simulink model "Navion_6DoF_YANG"  (Simulink 10.3)
settings: Solver=ode45  StartTime=0.0  StopTime=100.0  FixedStep=.01  MaxStep=.004  RelTol=1e-5  EnableMultiTasking=on
values from neighbouring files (symbols this model uses):
  ac = [0 0 0]    [Navion_Geom6dof.m]
  b = 44    [Navion_Geom6dof.m]
  cbar = 4+2/12    (= 4.16666666667)    [Navion_Geom6dof.m]
  cda2 = 0.33    [Navion_Geom6dof.m]
  cdo = 0.05    [Navion_Geom6dof.m]
  cg = [0 0 0]    [Navion_Geom6dof.m]
  cla = 4.44    [Navion_Geom6dof.m]
  cladot = 0    [Navion_Geom6dof.m]
  clb = -0.074    [Navion_Geom6dof.m]
  clda = -0.134    [Navion_Geom6dof.m]
  clde = 0.355    [Navion_Geom6dof.m]
  cldr = 0.107    [Navion_Geom6dof.m]
  clo = 0.41    [Navion_Geom6dof.m]
  clp = -0.410    (= -0.41)    [Navion_Geom6dof.m]
  clq = 3.8    [Navion_Geom6dof.m]
  clr = 0.107    [Navion_Geom6dof.m]
  cma = -0.683    [Navion_Geom6dof.m]
  cmadot = -4.36    [Navion_Geom6dof.m]
  cmde = -0.923    [Navion_Geom6dof.m]
  cmq = -9.96    [Navion_Geom6dof.m]
  cnb = 0.071    [Navion_Geom6dof.m]
  cnda = -0.0035    [Navion_Geom6dof.m]
  cndr = -0.072    [Navion_Geom6dof.m]
  cnp = -0.0575    [Navion_Geom6dof.m]
  cnr = -0.125    [Navion_Geom6dof.m]
  cyb = -0.564    [Navion_Geom6dof.m]
  cydr = 0.157    [Navion_Geom6dof.m]
  initalt = 6000    [Navion_Geom6dof.m]
  initbank = 0    [Navion_Geom6dof.m]
  initeast = 0    [Navion_Geom6dof.m]
  inithead = 0    [Navion_Geom6dof.m]
  initnorth = 0    [Navion_Geom6dof.m]
  initp = 0    [Navion_Geom6dof.m]
  initpitch = initw/initu    (= -0.0290599038041)    [Navion_Geom6dof.m]
  initq = 0    [Navion_Geom6dof.m]
  initr = 0    [Navion_Geom6dof.m]
  initu = 228.7    [Navion_Geom6dof.m]
  initv = 0    [Navion_Geom6dof.m]
  initw = -6.646    [Navion_Geom6dof.m]
  jx = 1048    [Navion_Geom6dof.m]
  jxz = 0    [Navion_Geom6dof.m]
  jy = 3000    [Navion_Geom6dof.m]
  jz = 3500    [Navion_Geom6dof.m]
  Pos_L = [95.46/12-3.882,5.1875,0]    [Navion_Geom6dof.m]
  Pos_R = [95.46/12,-5.1875,0]    [Navion_Geom6dof.m]
  sw = 175.3    [Navion_Geom6dof.m]
  Vect_L = [0.998,-0.057,0.017]    [Navion_Geom6dof.m]
  Vect_R = [0.998,0.057,0.017]    [Navion_Geom6dof.m]
  weight = 3695    [Navion_Geom6dof.m]
undefined symbols (not defined in the file or in its folder): BHP_A, BHP_B, CP_norm, Pr_Alt, PropEff_norm
libraries: simulink_extras x4, aerolibatmos2 x2
(part 2 of 2)

== system Navion_6DoF_YANG/Aircraft_Dynamics/Aerodynamics/Aero Forces and Moments/Aerodynamic Forces/Body to Wind ==
  note: This transforms any arbitrary vector from body axis to wind axis.
      | Page 63  Stevens and Lewis
  Alpha : Inport
  Beta : Inport  Port=2
  -ca sb : Fcn  Expr=-1 * cos(u[1]) * sin(u[2])
  -sa : Fcn  Expr=-1 * sin(u[1])
  -sa sb : Fcn  Expr="-1 * sin(u[1])  * sin(u[2])"
  Fcn8 : Fcn  Expr=cos(u[1])
  Matrix Concatenation : Concatenate  NumInputs=3  Mode=Multidimensional array
  Matrix Concatenation1 : Concatenate  NumInputs=3  Mode=Multidimensional array
  Matrix Concatenation2 : Concatenate  NumInputs=3  Mode=Multidimensional array  ConcatenateDimension=2
  Matrix Concatenation3 : Concatenate  NumInputs=3  Mode=Multidimensional array
  Mux1 : Mux  Inputs=2
  ca cb : Fcn  Expr="cos(u[1]) *  cos(u[2])"
  cb : Fcn  Expr=cos(u[2])
  sa cb : Fcn  Expr=sin(u[1]) * cos(u[2])
  sb : Fcn  Expr=sin(u[2])
  zero : Fcn  Expr=u[1] * 0
  Smatrix : Outport
  wires:
  Matrix Concatenation/1 -> Matrix Concatenation2/1
  Matrix Concatenation1/1 -> Matrix Concatenation2/2
  Matrix Concatenation3/1 -> Matrix Concatenation2/3
  -ca sb/1 -> Matrix Concatenation/2
  ca cb/1 -> Matrix Concatenation/1
  -sa/1 -> Matrix Concatenation/3
  zero/1 -> Matrix Concatenation1/3
  sb/1 -> Matrix Concatenation1/1
  cb/1 -> Matrix Concatenation1/2
  sa cb/1 -> Matrix Concatenation3/1
  -sa sb/1 -> Matrix Concatenation3/2
  Fcn8/1 -> Matrix Concatenation3/3
  Mux1/1 -> ca cb/1, -ca sb/1, -sa/1, sb/1, cb/1, zero/1, sa cb/1, -sa sb/1, Fcn8/1
  Alpha/1 -> Mux1/1
  Beta/1 -> Mux1/2
  Matrix Concatenation2/1 -> Smatrix/1

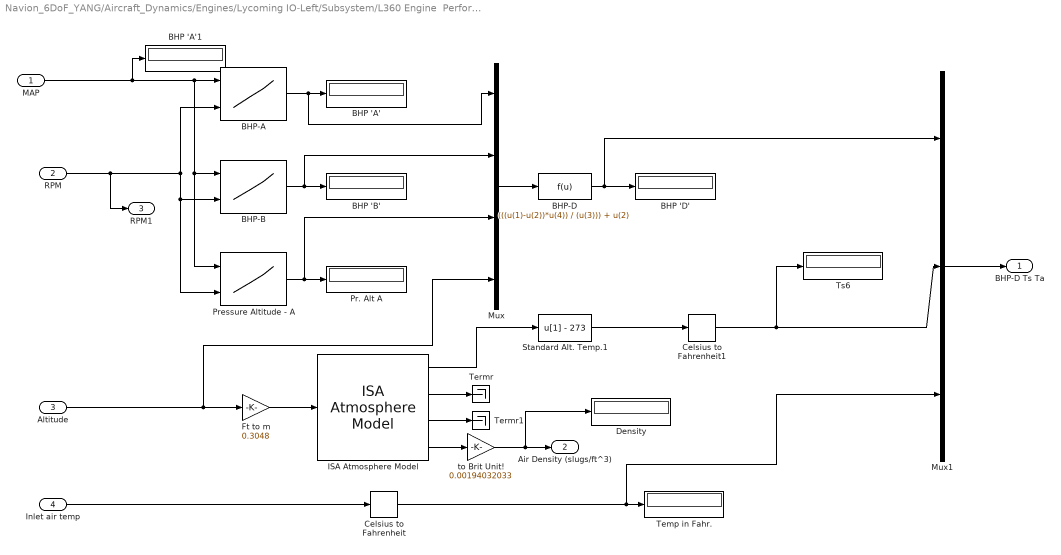
== system Navion_6DoF_YANG/Aircraft_Dynamics/Engines/Lycoming IO-Left/Subsystem/L360 Engine  Performance Data ==
  MAP : Inport
  RPM : Inport  Port=2
  Altitude : Inport  Port=3
  Inlet air temp : Inport  Port=4
  BHP 'A' : Display
  BHP 'A'1 : Display
  BHP 'B' : Display
  BHP 'D' : Display
  BHP-A : Lookup2D  RowIndex=MAP  ColumnIndex=RPM  Table=BHP_A  LookUpMeth=Interpolation-Use End Values
  BHP-B : Lookup2D  RowIndex=MAP  ColumnIndex=RPM  Table=BHP_B  LookUpMeth=Interpolation-Use End Values
  BHP-D : Fcn  Expr=(((u(1)-u(2))*u(4)) / (u(3))) + u(2)
  Celsius to Fahrenheit : simulink_extras/Transformations/Celsius to Fahrenheit
      settings: SourceProductBaseCode=SL
  Celsius to Fahrenheit1 : simulink_extras/Transformations/Celsius to Fahrenheit
      settings: SourceProductBaseCode=SL
  Density : Display
  Ft to m : Gain  Gain=0.3048
  ISA Atmosphere Model : aerolibatmos2/ISA Atmosphere Model  custom=off  g=9.80665  gamma=1.4  R=287.0531  L=0.0065  h_trop=11000  h_strat=20000  rho0=1.225  P0=101325  T0=288.15  h0=0
  Mux : Mux
  Mux1 : Mux  Inputs=3
  Pr. Alt A : Display
  Pressure Altitude - A : Lookup2D  RowIndex=MAP  ColumnIndex=RPM  Table=Pr_Alt  LookUpMeth=Interpolation-Use End Values
  Standard Alt. Temp.1 : Fcn  Expr=u[1] - 273
  Temp in Fahr. : Display
  Termr : Terminator
  Termr1 : Terminator
  Ts6 : Display
  to Brit Unit! : Gain  Gain=0.00194032033
  BHP-D Ts Ta : Outport
  Air Density (slugs/ft^3) : Outport  Port=2
  RPM1 : Outport  Port=3
  wires:
  MAP/1 -> BHP 'A'1/1, Pressure Altitude - A/1, BHP-B/1, BHP-A/1
  ISA Atmosphere Model/1 -> Standard Alt. Temp.1/1
  to Brit Unit!/1 -> Density/1, Air Density (slugs/ft^3)/1
  ISA Atmosphere Model/4 -> to Brit Unit!/1
  Altitude/1 -> Ft to m/1, Mux/4
  ISA Atmosphere Model/3 -> Termr1/1
  ISA Atmosphere Model/2 -> Termr/1
  Celsius to Fahrenheit1/1 -> Ts6/1, Mux1/2
  Standard Alt. Temp.1/1 -> Celsius to Fahrenheit1/1
  Ft to m/1 -> ISA Atmosphere Model/1
  Mux1/1 -> BHP-D Ts Ta/1
  Celsius to Fahrenheit/1 -> Temp in Fahr./1, Mux1/3
  Inlet air temp/1 -> Celsius to Fahrenheit/1
  BHP-D/1 -> Mux1/1, BHP 'D'/1
  Mux/1 -> BHP-D/1
  Pressure Altitude - A/1 -> Mux/3, Pr. Alt A/1
  BHP-A/1 -> Mux/1, BHP 'A'/1
  BHP-B/1 -> Mux/2, BHP 'B'/1
  RPM/1 -> RPM1/1, Pressure Altitude - A/2, BHP-B/2, BHP-A/2

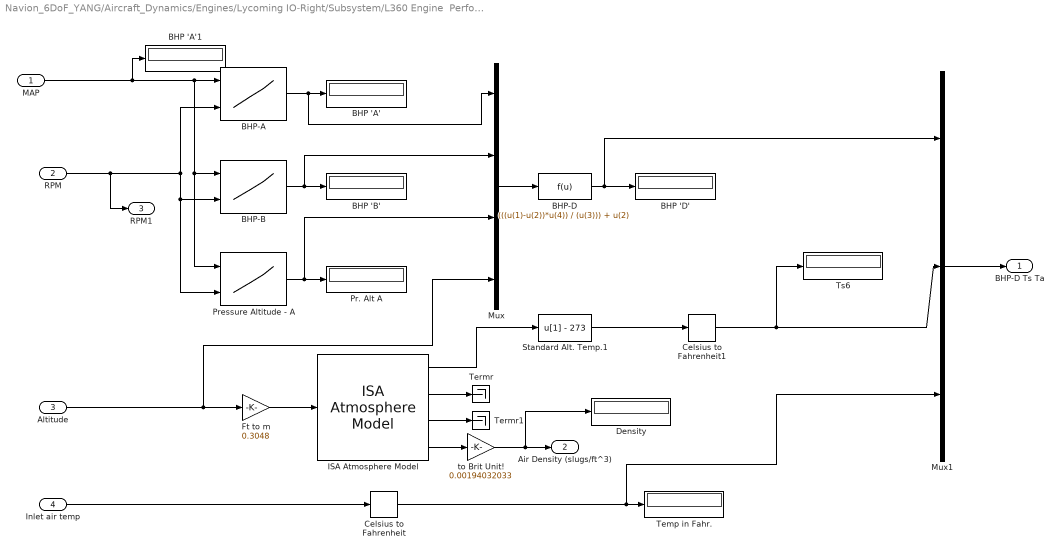
== system Navion_6DoF_YANG/Aircraft_Dynamics/Engines/Lycoming IO-Right/Subsystem/L360 Engine  Performance Data ==
  MAP : Inport
  RPM : Inport  Port=2
  Altitude : Inport  Port=3
  Inlet air temp : Inport  Port=4
  BHP 'A' : Display
  BHP 'A'1 : Display
  BHP 'B' : Display
  BHP 'D' : Display
  BHP-A : Lookup2D  RowIndex=MAP  ColumnIndex=RPM  Table=BHP_A  LookUpMeth=Interpolation-Use End Values
  BHP-B : Lookup2D  RowIndex=MAP  ColumnIndex=RPM  Table=BHP_B  LookUpMeth=Interpolation-Use End Values
  BHP-D : Fcn  Expr=(((u(1)-u(2))*u(4)) / (u(3))) + u(2)
  Celsius to Fahrenheit : simulink_extras/Transformations/Celsius to Fahrenheit
      settings: SourceProductBaseCode=SL
  Celsius to Fahrenheit1 : simulink_extras/Transformations/Celsius to Fahrenheit
      settings: SourceProductBaseCode=SL
  Density : Display
  Ft to m : Gain  Gain=0.3048
  ISA Atmosphere Model : aerolibatmos2/ISA Atmosphere Model  custom=off  g=9.80665  gamma=1.4  R=287.0531  L=0.0065  h_trop=11000  h_strat=20000  rho0=1.225  P0=101325  T0=288.15  h0=0
  Mux : Mux
  Mux1 : Mux  Inputs=3
  Pr. Alt A : Display
  Pressure Altitude - A : Lookup2D  RowIndex=MAP  ColumnIndex=RPM  Table=Pr_Alt  LookUpMeth=Interpolation-Use End Values
  Standard Alt. Temp.1 : Fcn  Expr=u[1] - 273
  Temp in Fahr. : Display
  Termr : Terminator
  Termr1 : Terminator
  Ts6 : Display
  to Brit Unit! : Gain  Gain=0.00194032033
  BHP-D Ts Ta : Outport
  Air Density (slugs/ft^3) : Outport  Port=2
  RPM1 : Outport  Port=3
  wires:
  MAP/1 -> BHP 'A'1/1, Pressure Altitude - A/1, BHP-B/1, BHP-A/1
  ISA Atmosphere Model/1 -> Standard Alt. Temp.1/1
  to Brit Unit!/1 -> Density/1, Air Density (slugs/ft^3)/1
  ISA Atmosphere Model/4 -> to Brit Unit!/1
  Altitude/1 -> Ft to m/1, Mux/4
  ISA Atmosphere Model/3 -> Termr1/1
  ISA Atmosphere Model/2 -> Termr/1
  Celsius to Fahrenheit1/1 -> Ts6/1, Mux1/2
  Standard Alt. Temp.1/1 -> Celsius to Fahrenheit1/1
  Ft to m/1 -> ISA Atmosphere Model/1
  Mux1/1 -> BHP-D Ts Ta/1
  Celsius to Fahrenheit/1 -> Temp in Fahr./1, Mux1/3
  Inlet air temp/1 -> Celsius to Fahrenheit/1
  BHP-D/1 -> Mux1/1, BHP 'D'/1
  Mux/1 -> BHP-D/1
  Pressure Altitude - A/1 -> Mux/3, Pr. Alt A/1
  BHP-A/1 -> Mux/1, BHP 'A'/1
  BHP-B/1 -> Mux/2, BHP 'B'/1
  RPM/1 -> RPM1/1, Pressure Altitude - A/2, BHP-B/2, BHP-A/2

== matlab function Aircraft_Dynamics/Engines/Lycoming IO-Left/Prop Efficiency with Cp input/Embedded MATLAB Function Retrieving Pich Angle ==
  data: CP input double; j input double; CP_norm input double; Pitch output double
function Pitch   =  fcn(CP, j, CP_norm)
%#eml

proppitch= [15 20 25 30 35 40];
tempJ = 0;
tempCP = 0;
Jindex = 1;
CPindex = 1;
% j = 0.4;
% CP = 0.22;

i=0;
for i=1:size(CP_norm,1)
    if j > CP_norm(i,1)
        
        tempJ = CP_norm(i,1);
        Jindex = i;
    end
end
for a=1:size(CP_norm,2)
    if CP > CP_norm(Jindex,a)
        tempCP = CP_norm(a,1);
        CPindex = a;
    end
end

if (CPindex ~= 0 && Jindex ~= 0)
    if (CPindex) == 7;
        Pitch = 40 ; 
    else
        if CPindex == 1
            Pitch =15;
        else
            Pitch = interp1(CP_norm(Jindex,CPindex:CPindex+1),proppitch(CPindex-1:CPindex),CP);
        end
        
    end
else
    Pitch = 15;

end
return

== matlab function Aircraft_Dynamics/Engines/Lycoming IO-Right/Prop Efficiency with Cp input/Embedded MATLAB Function Retrieving Pich Angle ==
  data: CP input double; j input double; CP_norm input double; Pitch output double
function Pitch   =  fcn(CP, j, CP_norm)
%#eml

proppitch= [15 20 25 30 35 40];
tempJ = 0;
tempCP = 0;
Jindex = 1;
CPindex = 1;
% j = 0.4;
% CP = 0.22;

i=0;
for i=1:size(CP_norm,1)
    if j > CP_norm(i,1)
        
        tempJ = CP_norm(i,1);
        Jindex = i;
    end
end
for a=1:size(CP_norm,2)
    if CP > CP_norm(Jindex,a)
        tempCP = CP_norm(a,1);
        CPindex = a;
    end
end

if (CPindex ~= 0 && Jindex ~= 0)
    if (CPindex) == 7;
        Pitch = 40 ; 
    else
        if CPindex == 1
            Pitch =15;
        else
            Pitch = interp1(CP_norm(Jindex,CPindex:CPindex+1),proppitch(CPindex-1:CPindex),CP);
        end
        
    end
else
    Pitch = 15;

end
return
